simulink model "BOZ"  (R2021a)
settings: Solver=FixedStepAuto  StartTime=0.0  StopTime=3  RelTol=1e-3
settings Model: Creator=xpess  LastModifiedBy=xpess

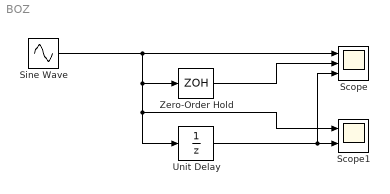
== system BOZ ==
  Scope : Scope  NumInputPorts=3
  Scope1 : Scope  NumInputPorts=2
  Sine Wave : Sin  Frequency=2*pi  SampleTime=0.01
  Unit Delay : UnitDelay  SampleTime=.05  HasFrameUpgradeWarning=on
  Zero-Order Hold : ZeroOrderHold  SampleTime=0.05
  wires:
  Sine Wave/1 -> Unit Delay/1, Scope1/1, Zero-Order Hold/1, Scope/1
  Zero-Order Hold/1 -> Scope/2
  Unit Delay/1 -> Scope/3, Scope1/2
